simulink library "lib_Convection_FCHorizCyl"  (R2015a)
settings: Solver=ode45  StartTime=0.0  StopTime=10.0  RelTol=1e-3
libraries: simulink x9, lib_GenTools_MinMax x1
settings Model: Creator=jlkratz  LastModifiedBy=jlkratz

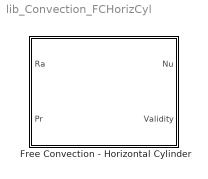
== system lib_Convection_FCHorizCyl ==
  Free Convection - Horizontal Cylinder : Subsystem  mask(TSAT: Horizontal Cylinder Free Convection){Corr_M=Correlation 1 - Morgan}
      mask prompts: Corr_M "Corr_M - Correlation Choice"
      mask help: This block estimates the average Nusselt number of a free convecting flow about a horizontal isothermal cylinder. This block allows the application of two different correlations. The first is a set of equations developed by Morgan, each of which is valid over a different Rayliegh number (Ra) range. The second is a single correlation developed by Churchil and Chu that is valid over a wide range of Rayliegh numbers. The Rayliegh number should be calculated using the diameter of the cylinder as the characteristic length. Note that all fluid properrties should be evaluated at film temperature (average of the bulk fluid and surface temperatures).
      mask Help: web(which('Convection_TSAT_FCHorizCyl.html'),'-helpbrowser')
      mask TypeOptions Corr_M: Correlation 1 - Morgan | Correlation 2 - Churchill and Chu
      mask DialogControl Container6 Prompt: Parameters

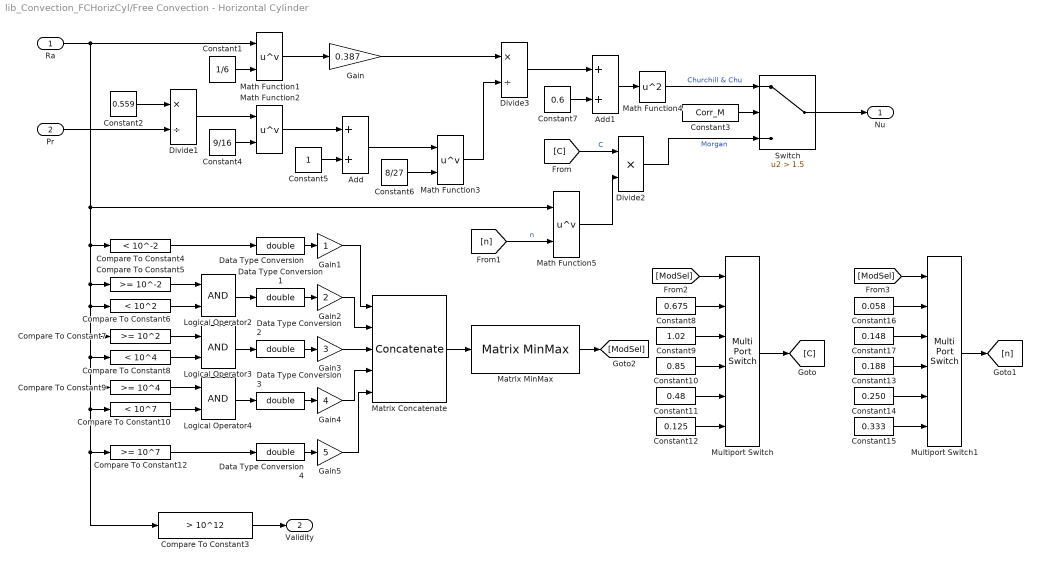
== system lib_Convection_FCHorizCyl/Free Convection - Horizontal Cylinder ==
  Ra : Inport
  Pr : Inport  Port=2
  Add : Sum
  Add1 : Sum
  Compare To Constant10 : simulink/Logic and Bit Operations/Compare To Constant  relop=<  const=10^7  OutDataTypeStr=boolean
  Compare To Constant12 : simulink/Logic and Bit Operations/Compare To Constant  relop=>=  const=10^7  OutDataTypeStr=boolean
  Compare To Constant3 : simulink/Logic and Bit Operations/Compare To Constant  relop=>  const=10^12  OutDataTypeStr=boolean
  Compare To Constant4 : simulink/Logic and Bit Operations/Compare To Constant  relop=<  const=10^-2  OutDataTypeStr=boolean
  Compare To Constant5 : simulink/Logic and Bit Operations/Compare To Constant  relop=>=  const=10^-2  OutDataTypeStr=boolean
  Compare To Constant6 : simulink/Logic and Bit Operations/Compare To Constant  relop=<  const=10^2  OutDataTypeStr=boolean
  Compare To Constant7 : simulink/Logic and Bit Operations/Compare To Constant  relop=>=  const=10^2  OutDataTypeStr=boolean
  Compare To Constant8 : simulink/Logic and Bit Operations/Compare To Constant  relop=<  const=10^4  OutDataTypeStr=boolean
  Compare To Constant9 : simulink/Logic and Bit Operations/Compare To Constant  relop=>=  const=10^4  OutDataTypeStr=boolean
  Constant1 : Constant  Value=1/6
  Constant10 : Constant  Value=0.85
  Constant11 : Constant  Value=0.48
  Constant12 : Constant  Value=0.125
  Constant13 : Constant  Value=0.188
  Constant14 : Constant  Value=0.250
  Constant15 : Constant  Value=0.333
  Constant16 : Constant  Value=0.058
  Constant17 : Constant  Value=0.148
  Constant2 : Constant  Value=0.559
  Constant3 : Constant  Value=Corr_M
  Constant4 : Constant  Value=9/16
  Constant5 : Constant
  Constant6 : Constant  Value=8/27
  Constant7 : Constant  Value=0.6
  Constant8 : Constant  Value=0.675
  Constant9 : Constant  Value=1.02
  Data Type Conversion{,1..4} (5 alike) : DataTypeConversion  OutDataTypeStr=double
  Divide1 : Product  Inputs=*/
  Divide2 : Product  Inputs=**
  Divide3 : Product  Inputs=*/
  Gain : Gain  Gain=0.387
  Gain1 : Gain
  Gain2 : Gain  Gain=2
  Gain3 : Gain  Gain=3
  Gain4 : Gain  Gain=4
  Gain5 : Gain  Gain=5
  Logical Operator2 : Logic  AllPortsSameDT=off  OutDataTypeStr=boolean
  Logical Operator3 : Logic  AllPortsSameDT=off  OutDataTypeStr=boolean
  Logical Operator4 : Logic  AllPortsSameDT=off  OutDataTypeStr=boolean
  Math Function{1..3,5} (4 alike) : Math  Operator=pow  SaturateOnIntegerOverflow=on
  Math Function4 : Math  Operator=square  SaturateOnIntegerOverflow=on
  Matrix Concatenate : Concatenate  NumInputs=5  Mode=Multidimensional array  ConcatenateDimension=2
  Matrix MinMax : lib_GenTools_MinMax/Matrix MinMax  rows_M=on  cols_M=off  all_M=off  minmax_M=off  BN_M=gcb
  Multiport Switch : MultiPortSwitch  Inputs=5
  Multiport Switch1 : MultiPortSwitch  Inputs=5
  Switch : Switch  Criteria=u2 > Threshold  Threshold=1.5
  Nu : Outport
  Validity : Outport  Port=2
  wires:
  Ra/1 -> Math Function1/1, Math Function5/1, Compare To Constant3/1, Compare To Constant12/1, Compare To Constant10/1, Compare To Constant9/1, Compare To Constant8/1, Compare To Constant7/1, Compare To Constant6/1, Compare To Constant5/1, Compare To Constant4/1
  Compare To Constant12/1 -> Data Type Conversion4/1
  Logical Operator4/1 -> Data Type Conversion3/1
  Logical Operator3/1 -> Data Type Conversion2/1
  Logical Operator2/1 -> Data Type Conversion1/1
  Compare To Constant4/1 -> Data Type Conversion/1
  Compare To Constant9/1 -> Logical Operator4/1
  Compare To Constant10/1 -> Logical Operator4/2
  Compare To Constant7/1 -> Logical Operator3/1
  Compare To Constant8/1 -> Logical Operator3/2
  Compare To Constant5/1 -> Logical Operator2/1
  Compare To Constant6/1 -> Logical Operator2/2
  Gain5/1 -> Matrix Concatenate/5
  Gain4/1 -> Matrix Concatenate/4
  Gain3/1 -> Matrix Concatenate/3
  Gain2/1 -> Matrix Concatenate/2
  Gain1/1 -> Matrix Concatenate/1
  Matrix Concatenate/1 -> Matrix MinMax/1
  Matrix MinMax/1 -> [ModSel]
  Data Type Conversion/1 -> Gain1/1
  Data Type Conversion1/1 -> Gain2/1
  Data Type Conversion2/1 -> Gain3/1
  Data Type Conversion3/1 -> Gain4/1
  Data Type Conversion4/1 -> Gain5/1
  [ModSel] -> Multiport Switch1/1
  [ModSel] -> Multiport Switch/1
  Multiport Switch/1 -> [C]
  Multiport Switch1/1 -> [n]
  Constant16/1 -> Multiport Switch1/2
  Constant17/1 -> Multiport Switch1/3
  Constant13/1 -> Multiport Switch1/4
  Constant14/1 -> Multiport Switch1/5
  Constant8/1 -> Multiport Switch/2
  Constant9/1 -> Multiport Switch/3
  Constant10/1 -> Multiport Switch/4
  Constant11/1 -> Multiport Switch/5
  Constant15/1 -> Multiport Switch1/6
  Constant12/1 -> Multiport Switch/6
  Constant3/1 -> Switch/2
  Switch/1 -> Nu/1
  Divide2/1 -> Switch/3  "Morgan"
  Math Function4/1 -> Switch/1  "Churchill & Chu"
  Math Function5/1 -> Divide2/2
  [n] -> Math Function5/2  "n"
  [C] -> Divide2/1  "C"
  Constant7/1 -> Add1/2
  Divide3/1 -> Add1/1
  Add1/1 -> Math Function4/1
  Math Function3/1 -> Divide3/2
  Gain/1 -> Divide3/1
  Constant6/1 -> Math Function3/2
  Add/1 -> Math Function3/1
  Constant5/1 -> Add/2
  Math Function2/1 -> Add/1
  Constant4/1 -> Math Function2/2
  Divide1/1 -> Math Function2/1
  Constant2/1 -> Divide1/1
  Math Function1/1 -> Gain/1
  Compare To Constant3/1 -> Validity/1
  Constant1/1 -> Math Function1/2
  Pr/1 -> Divide1/2
